simulink model "System_2"  (R2022b)
settings: Solver=VariableStepAuto  StartTime=0.0  StopTime=30  FixedStep=1e-3  MaxStep=1e-4  RelTol=1e-3
settings Model: Creator=Dongr  LastModifiedBy=Dong

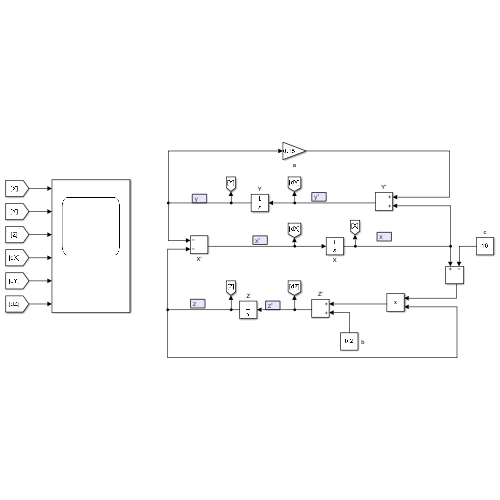
[thumbnail: Simulink's stored preview of the top-level diagram]
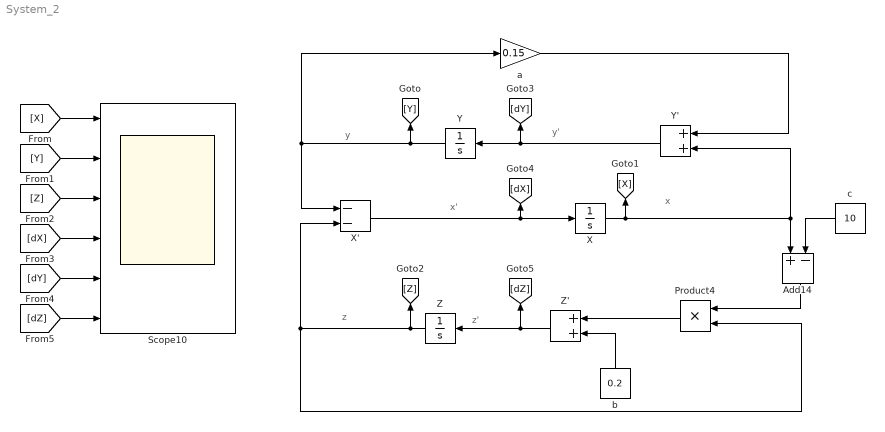
== system System_2 ==
  note: z'
  note: z
  note: x'
  note: y
  note: y'
  note: x
  Add14 : Sum  Inputs=+-
  Product4 : Product
  Scope10 : Scope  NumInputPorts=6
  X : Integrator
  X' : Sum  Inputs=--
  Y : Integrator
  Y' : Sum
  Z : Integrator
  Z' : Sum
  a : Gain  Gain=0.15
  b : Constant  Value=0.2
  c : Constant  Value=10
  wires:
  c/1 -> Add14/2
  Z'/1 -> [dZ], Z/1
  b/1 -> Z'/2
  Product4/1 -> Z'/1
  Add14/1 -> Product4/1
  Y/1 -> [Y], X'/1, a/1
  a/1 -> Y'/1
  Y'/1 -> Y/1, [dY]
  Z/1 -> [Z], Product4/2, X'/2
  X/1 -> [X], Add14/1, Y'/2
  X'/1 -> [dX], X/1
  [X] -> Scope10/1
  [Y] -> Scope10/2
  [Z] -> Scope10/3
  [dX] -> Scope10/4
  [dY] -> Scope10/5
  [dZ] -> Scope10/6
